simulink model "IP_Core_SS_Switch_and_PWM"  (R2018a)
settings: Solver=VariableStepAuto  StartTime=0.0  StopTime=0.05  RelTol=1e-3
values from neighbouring files (symbols this model uses):
  f_pwm_clk = 100e6    (= 100000000)    [Init_IP_Core.m]
  T_pwm_clk = 1/f_pwm_clk    (= 1e-08)    [Init_IP_Core.m]
libraries: hdlsllib x2
settings Model: Creator=BHK  LastModifiedBy=Wendel
settings OptimizationCC: BlockReduction=off  ConditionallyExecuteInputs=off  DefaultParameterBehavior=Inlined
settings DebuggingCC: AlgebraicLoopMsg=error
settings HardwareCC: ProdBitPerPointer=32  ProdBitPerSizeT=32  ProdBitPerPtrDiffT=32  ProdLargestAtomicFloat=None  ProdIntDivRoundTo=Undefined  ProdEndianess=Unspecified  ProdWordSize=32  ProdHWDeviceType=ASIC/FPGA->ASIC/FPGA  TargetBitPerPointer=64  TargetBitPerSizeT=64  TargetBitPerPtrDiffT=64  TargetLongLongMode=on  TargetIntDivRoundTo=Zero  TargetEndianess=LittleEndian  TargetWordSize=64  TargetHWDeviceType=Custom Processor->MATLAB Host Computer  ProdEqTarget=off

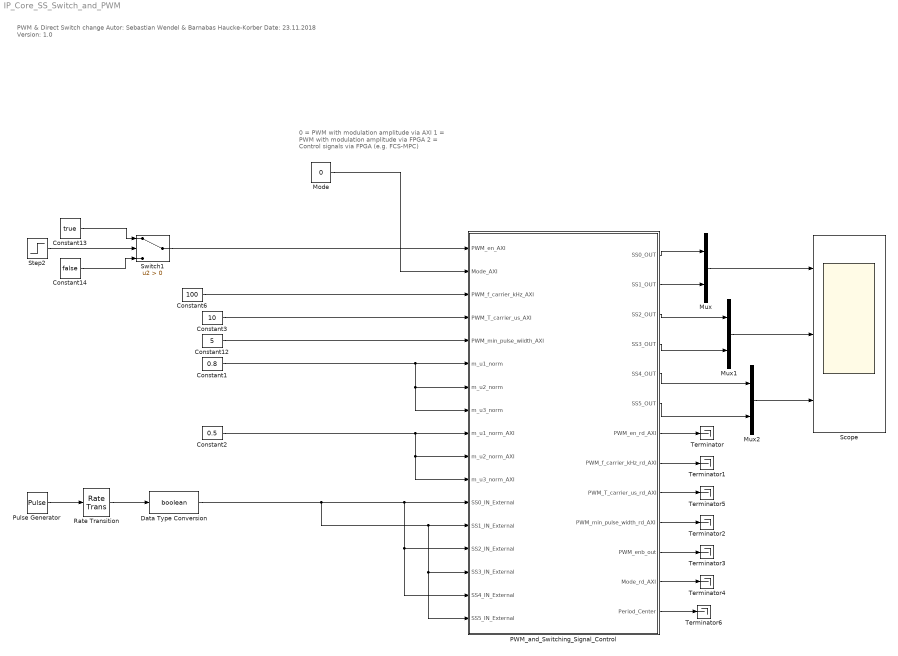
== system IP_Core_SS_Switch_and_PWM ==
  note: 0 = PWM with modulation amplitude via AXI
      | 1 = PWM with modulation amplitude via FPGA
      | 2 = Control signals via FPGA (e.g. FCS-MPC)
  note: PWM & Direct Switch change
      |
      | Autor: Sebastian Wendel & Barnabas Haucke-Korber
      | Date: 23.11.2018
      | Version: 1.0
  Constant1 : Constant  Value=0.8  OutDataTypeStr=fixdt(1,14,12)  SampleTime=T_pwm_clk
  Constant12 : Constant  Value=5  OutDataTypeStr=fixdt(0,8,0)  SampleTime=T_pwm_clk
  Constant13 : Constant  Value=true  SampleTime=T_pwm_clk
  Constant14 : Constant  Value=false  SampleTime=T_pwm_clk
  Constant2 : Constant  Value=0.5  OutDataTypeStr=fixdt(1,14,12)  SampleTime=T_pwm_clk
  Constant3 : Constant  Value=10  OutDataTypeStr=fixdt(0,8,0)  SampleTime=T_pwm_clk
  Constant6 : Constant  Value=100  OutDataTypeStr=fixdt(0,8,0)  SampleTime=T_pwm_clk
  Data Type Conversion : DataTypeConversion  OutDataTypeStr=boolean
  Mode : Constant  Value=0  OutDataTypeStr=fixdt(0,2,0)  SampleTime=T_pwm_clk
  Mux : Mux  Inputs=2
  Mux1 : Mux  Inputs=2
  Mux2 : Mux  Inputs=2
  PWM_and_Switching_Signal_Control : Subsystem  TreatAsAtomicUnit=on
  Pulse Generator : DiscretePulseGenerator  PulseType=Time based  Period=0.01  PulseWidth=5
  Rate Transition : RateTransition  OutPortSampleTime=T_pwm_clk
  Scope : Scope  NumInputPorts=3
  Step2 : Step  Time=0.002  SampleTime=T_pwm_clk
  Switch1 : Switch  Criteria=u2 > Threshold
  Terminator{,1..6} (7 alike) : Terminator
  wires:
  Step2/1 -> Switch1/2
  Constant13/1 -> Switch1/1
  Constant14/1 -> Switch1/3
  Switch1/1 -> PWM_and_Switching_Signal_Control/1(PWM_en_AXI)
  Mode/1 -> PWM_and_Switching_Signal_Control/2(Mode_AXI)
  Constant6/1 -> PWM_and_Switching_Signal_Control/3(PWM_f_carrier_kHz_AXI)
  Constant12/1 -> PWM_and_Switching_Signal_Control/5(PWM_min_pulse_wiidth_AXI)
  Constant1/1 -> PWM_and_Switching_Signal_Control/6(m_u1_norm), PWM_and_Switching_Signal_Control/8(m_u3_norm), PWM_and_Switching_Signal_Control/7(m_u2_norm)
  PWM_and_Switching_Signal_Control/7(PWM_en_rd_AXI) -> Terminator/1
  PWM_and_Switching_Signal_Control/8(PWM_f_carrier_kHz_rd_AXI) -> Terminator1/1
  PWM_and_Switching_Signal_Control/10(PWM_min_pulse_width_rd_AXI) -> Terminator2/1
  PWM_and_Switching_Signal_Control/11(PWM_enb_out) -> Terminator3/1
  PWM_and_Switching_Signal_Control/12(Mode_rd_AXI) -> Terminator4/1
  Constant2/1 -> PWM_and_Switching_Signal_Control/9(m_u1_norm_AXI), PWM_and_Switching_Signal_Control/10(m_u2_norm_AXI), PWM_and_Switching_Signal_Control/11(m_u3_norm_AXI)
  PWM_and_Switching_Signal_Control/1(SS0_OUT) -> Mux/1
  PWM_and_Switching_Signal_Control/2(SS1_OUT) -> Mux/2
  Mux/1 -> Scope/1
  PWM_and_Switching_Signal_Control/3(SS2_OUT) -> Mux1/1
  PWM_and_Switching_Signal_Control/4(SS3_OUT) -> Mux1/2
  PWM_and_Switching_Signal_Control/5(SS4_OUT) -> Mux2/1
  PWM_and_Switching_Signal_Control/6(SS5_OUT) -> Mux2/2
  Mux2/1 -> Scope/3
  Mux1/1 -> Scope/2
  Data Type Conversion/1 -> PWM_and_Switching_Signal_Control/17(SS5_IN_External), PWM_and_Switching_Signal_Control/15(SS3_IN_External), PWM_and_Switching_Signal_Control/13(SS1_IN_External), PWM_and_Switching_Signal_Control/16(SS4_IN_External), PWM_and_Switching_Signal_Control/14(SS2_IN_External), PWM_and_Switching_Signal_Control/12(SS0_IN_External)
  Constant3/1 -> PWM_and_Switching_Signal_Control/4(PWM_T_carrier_us_AXI)
  Rate Transition/1 -> Data Type Conversion/1
  Pulse Generator/1 -> Rate Transition/1
  PWM_and_Switching_Signal_Control/9(PWM_T_carrier_us_rd_AXI) -> Terminator5/1
  PWM_and_Switching_Signal_Control/13(Period_Center) -> Terminator6/1

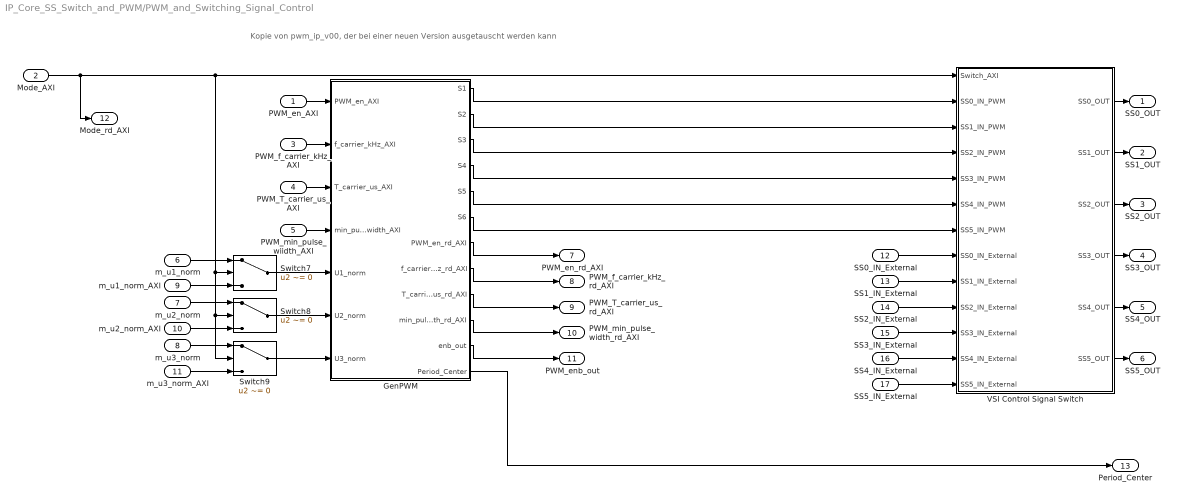
== system IP_Core_SS_Switch_and_PWM/PWM_and_Switching_Signal_Control ==
  note: Kopie von pwm_ip_v00, der bei einer neuen Version ausgetauscht werden kann
  PWM_en_AXI : Inport
  Mode_AXI : Inport  Port=2
  PWM_f_carrier_kHz_AXI : Inport  Port=3
  PWM_T_carrier_us_AXI : Inport  Port=4
  PWM_min_pulse_wiidth_AXI : Inport  Port=5
  m_u1_norm : Inport  Port=6
  m_u2_norm : Inport  Port=7
  m_u3_norm : Inport  Port=8
  m_u1_norm_AXI : Inport  Port=9
  m_u2_norm_AXI : Inport  Port=10
  m_u3_norm_AXI : Inport  Port=11
  SS0_IN_External : Inport  Port=12
  SS1_IN_External : Inport  Port=13
  SS2_IN_External : Inport  Port=14
  SS3_IN_External : Inport  Port=15
  SS4_IN_External : Inport  Port=16
  SS5_IN_External : Inport  Port=17
  GenPWM : Subsystem  TreatAsAtomicUnit=on
  Switch7 : Switch  Criteria=u2 ~= 0
  Switch8 : Switch  Criteria=u2 ~= 0
  Switch9 : Switch  Criteria=u2 ~= 0
  VSI Control Signal Switch : Subsystem
  SS0_OUT : Outport
  SS1_OUT : Outport  Port=2
  SS2_OUT : Outport  Port=3
  SS3_OUT : Outport  Port=4
  SS4_OUT : Outport  Port=5
  SS5_OUT : Outport  Port=6
  PWM_en_rd_AXI : Outport  Port=7
  PWM_f_carrier_kHz_rd_AXI : Outport  Port=8
  PWM_T_carrier_us_rd_AXI : Outport  Port=9
  PWM_min_pulse_width_rd_AXI : Outport  Port=10
  PWM_enb_out : Outport  Port=11
  Mode_rd_AXI : Outport  Port=12
  Period_Center : Outport  Port=13
  wires:
  VSI Control Signal Switch/1(SS0_OUT) -> SS0_OUT/1
  Mode_AXI/1 -> Mode_rd_AXI/1, VSI Control Signal Switch/1(Switch_AXI), Switch7/2, Switch9/2, Switch8/2
  GenPWM/4(S4) -> VSI Control Signal Switch/5(SS3_IN_PWM)
  PWM_f_carrier_kHz_AXI/1 -> GenPWM/2(f_carrier_kHz_AXI)
  GenPWM/2(S2) -> VSI Control Signal Switch/3(SS1_IN_PWM)
  SS1_IN_External/1 -> VSI Control Signal Switch/9(SS1_IN_External)
  GenPWM/3(S3) -> VSI Control Signal Switch/4(SS2_IN_PWM)
  GenPWM/5(S5) -> VSI Control Signal Switch/6(SS4_IN_PWM)
  GenPWM/6(S6) -> VSI Control Signal Switch/7(SS5_IN_PWM)
  VSI Control Signal Switch/6(SS5_OUT) -> SS5_OUT/1
  GenPWM/1(S1) -> VSI Control Signal Switch/2(SS0_IN_PWM)
  GenPWM/11(enb_out) -> PWM_enb_out/1
  VSI Control Signal Switch/3(SS2_OUT) -> SS2_OUT/1
  SS3_IN_External/1 -> VSI Control Signal Switch/11(SS3_IN_External)
  SS0_IN_External/1 -> VSI Control Signal Switch/8(SS0_IN_External)
  VSI Control Signal Switch/2(SS1_OUT) -> SS1_OUT/1
  SS4_IN_External/1 -> VSI Control Signal Switch/12(SS4_IN_External)
  PWM_en_AXI/1 -> GenPWM/1(PWM_en_AXI)
  SS5_IN_External/1 -> VSI Control Signal Switch/13(SS5_IN_External)
  VSI Control Signal Switch/5(SS4_OUT) -> SS4_OUT/1
  PWM_min_pulse_wiidth_AXI/1 -> GenPWM/4(min_pulse_width_AXI)
  SS2_IN_External/1 -> VSI Control Signal Switch/10(SS2_IN_External)
  VSI Control Signal Switch/4(SS3_OUT) -> SS3_OUT/1
  Switch9/1 -> GenPWM/7(U3_norm)
  m_u1_norm_AXI/1 -> Switch7/3
  m_u1_norm/1 -> Switch7/1
  m_u2_norm/1 -> Switch8/1
  m_u2_norm_AXI/1 -> Switch8/3
  m_u3_norm/1 -> Switch9/1
  m_u3_norm_AXI/1 -> Switch9/3
  GenPWM/7(PWM_en_rd_AXI) -> PWM_en_rd_AXI/1
  GenPWM/8(f_carrier_kHz_rd_AXI) -> PWM_f_carrier_kHz_rd_AXI/1
  GenPWM/10(min_pulse_width_rd_AXI) -> PWM_min_pulse_width_rd_AXI/1
  GenPWM/9(T_carrier_us_rd_AXI) -> PWM_T_carrier_us_rd_AXI/1
  Switch8/1 -> GenPWM/6(U2_norm)
  Switch7/1 -> GenPWM/5(U1_norm)
  PWM_T_carrier_us_AXI/1 -> GenPWM/3(T_carrier_us_AXI)
  GenPWM/12(Period_Center) -> Period_Center/1

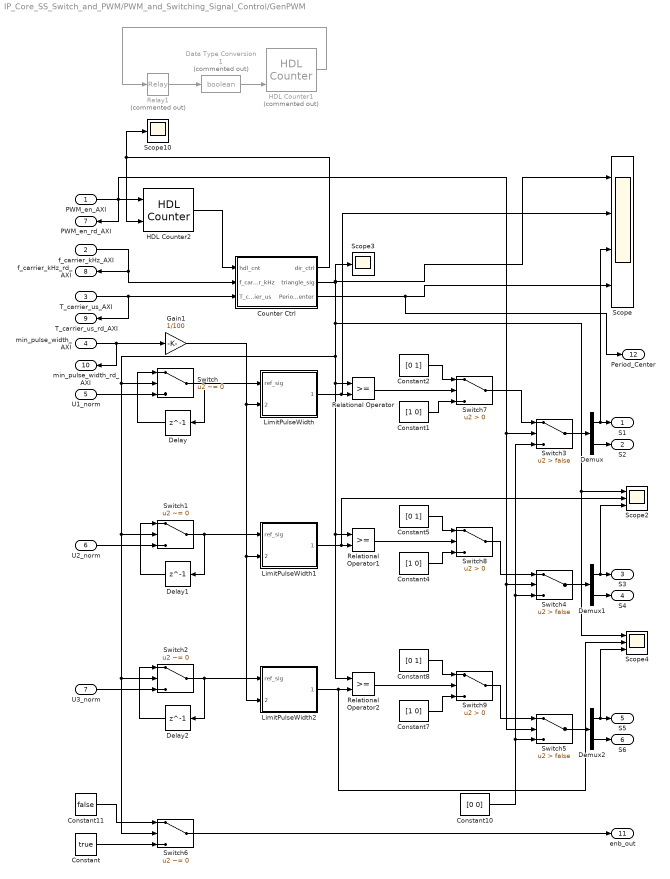
== system IP_Core_SS_Switch_and_PWM/PWM_and_Switching_Signal_Control/GenPWM ==
  PWM_en_AXI : Inport
  f_carrier_kHz_AXI : Inport  Port=2
  T_carrier_us_AXI : Inport  Port=3
  min_pulse_width_AXI : Inport  Port=4
  U1_norm : Inport  Port=5
  U2_norm : Inport  Port=6
  U3_norm : Inport  Port=7
  Constant : Constant  Value=true  SampleTime=T_pwm_clk
  Constant1 : Constant  Value=[1 0]  OutDataTypeStr=fixdt(0,1,0)  SampleTime=T_pwm_clk
  Constant10 : Constant  Value=[0 0]  OutDataTypeStr=fixdt(0,1,0)  SampleTime=T_pwm_clk
  Constant11 : Constant  Value=false  SampleTime=T_pwm_clk
  Constant2 : Constant  Value=[0 1]  OutDataTypeStr=fixdt(0,1,0)  SampleTime=T_pwm_clk
  Constant4 : Constant  Value=[1 0]  OutDataTypeStr=fixdt(0,1,0)  SampleTime=T_pwm_clk
  Constant5 : Constant  Value=[0 1]  OutDataTypeStr=fixdt(0,1,0)  SampleTime=T_pwm_clk
  Constant7 : Constant  Value=[1 0]  OutDataTypeStr=fixdt(0,1,0)  SampleTime=T_pwm_clk
  Constant8 : Constant  Value=[0 1]  OutDataTypeStr=fixdt(0,1,0)  SampleTime=T_pwm_clk
  Counter Ctrl : Subsystem
  Data Type Conversion1 : DataTypeConversion  Commented=on  OutDataTypeStr=boolean
  Delay : Delay  DelayLength=1
  Delay1 : Delay  DelayLength=1
  Delay2 : Delay  DelayLength=1
  Demux : Demux  Outputs=2
  Demux1 : Demux  Outputs=2
  Demux2 : Demux  Outputs=2
  Gain1 : Gain  Gain=1/100  OutDataTypeStr=fixdt(1,18,10)
  HDL Counter1 : hdlsllib/Sources/HDL Counter  Commented=on  CountType=Free running  CountInit=0  CountStep=1  CountMax=100  CountFromType=Initial value  CountFrom=0  CountResetPort=on  CountLoadPort=off  CountEnbPort=on  CountDirPort=on  CountDataType=Signed  CountWordLen=8  CountFracLen=0  CountSampTime=Ts
      settings: SourceProductBaseCode=HD
  HDL Counter2 : hdlsllib/Sources/HDL Counter  CountType=Free running  CountInit=0  CountStep=1  CountMax=100  CountFromType=Initial value  CountFrom=0  CountResetPort=off  CountLoadPort=off  CountEnbPort=on  CountDirPort=on  CountDataType=Unsigned  CountWordLen=20  CountFracLen=0  CountSampTime=1
      settings: SourceProductBaseCode=HD
  LimitPulseWidth : Subsystem
  LimitPulseWidth1 : Subsystem
  LimitPulseWidth2 : Subsystem
  Relational Operator : RelationalOperator  OutDataTypeStr=boolean  RndMeth=Nearest
  Relational Operator1 : RelationalOperator  OutDataTypeStr=boolean  RndMeth=Nearest
  Relational Operator2 : RelationalOperator  OutDataTypeStr=boolean  RndMeth=Nearest
  Relay1 : Relay  Commented=on  OnSwitchValue=100  OffSwitchValue=0  OnOutputValue=0  OffOutputValue=1
  Scope : Scope  NumInputPorts=4
  Scope10 : Scope
  Scope2 : Scope  NumInputPorts=3
  Scope3 : Scope
  Scope4 : Scope  NumInputPorts=3
  Switch{,1..2,6} (4 alike) : Switch  Criteria=u2 ~= 0
  Switch3 : Switch  Criteria=u2 > Threshold  Threshold=false
  Switch4 : Switch  Criteria=u2 > Threshold  Threshold=false
  Switch5 : Switch  Criteria=u2 > Threshold  Threshold=false
  Switch7 : Switch  Criteria=u2 > Threshold
  Switch8 : Switch  Criteria=u2 > Threshold
  Switch9 : Switch  Criteria=u2 > Threshold
  S1 : Outport
  S2 : Outport  Port=2
  S3 : Outport  Port=3
  S4 : Outport  Port=4
  S5 : Outport  Port=5
  S6 : Outport  Port=6
  PWM_en_rd_AXI : Outport  Port=7
  f_carrier_kHz_rd_AXI : Outport  Port=8
  T_carrier_us_rd_AXI : Outport  Port=9
  min_pulse_width_rd_AXI : Outport  Port=10
  enb_out : Outport  Port=11
  Period_Center : Outport  Port=12
  wires:
  Constant7/1 -> Switch9/3
  Demux2/2 -> S6/1
  Constant8/1 -> Switch9/1
  Relational Operator2/1 -> Switch9/2
  Switch9/1 -> Switch5/1
  Demux/2 -> S2/1
  Relational Operator/1 -> Switch7/2
  Demux1/2 -> S4/1
  Constant5/1 -> Switch8/1
  Relational Operator1/1 -> Switch8/2
  Constant4/1 -> Switch8/3
  Constant1/1 -> Switch7/3
  Constant2/1 -> Switch7/1
  LimitPulseWidth/1(ref_sig_limit) -> Scope/2, Relational Operator/2
  LimitPulseWidth1/1(ref_sig_limit) -> Scope2/2, Relational Operator1/2
  LimitPulseWidth2/1(ref_sig_limit) -> Scope4/2, Relational Operator2/2
  Counter Ctrl/2(triangle_sig) -> Relational Operator2/1, Relational Operator1/1, Relational Operator/1, Switch6/2, Switch2/2, Switch1/2, Switch/2, Scope4/1, Scope2/1, Scope3/1, Scope/1
  PWM_en_AXI/1 -> Switch3/2, Switch5/2, Switch4/2, PWM_en_rd_AXI/1, HDL Counter2/1
  Delay/1 -> Switch/1
  Delay1/1 -> Switch1/1
  Delay2/1 -> Switch2/1
  Switch5/1 -> Demux2/1
  Switch8/1 -> Switch4/1
  Switch4/1 -> Demux1/1
  Switch3/1 -> Demux/1
  Constant10/1 -> Switch5/3, Switch4/3, Switch3/3
  U1_norm/1 -> Switch/3
  U3_norm/1 -> Switch2/3
  U2_norm/1 -> Switch1/3
  Counter Ctrl/1(dir_ctrl) -> HDL Counter2/2, Scope10/1
  HDL Counter2/1 -> Counter Ctrl/1(hdl_cnt)
  f_carrier_kHz_AXI/1 -> f_carrier_kHz_rd_AXI/1, Counter Ctrl/2(f_carrier_kHz)
  Relay1/1 -> Data Type Conversion1/1
  Data Type Conversion1/1 -> HDL Counter1/3
  HDL Counter1/1 -> Relay1/1
  Switch/1 -> LimitPulseWidth/1(ref_sig), Delay/1
  Switch1/1 -> LimitPulseWidth1/1(ref_sig), Delay1/1
  Switch2/1 -> LimitPulseWidth2/1(ref_sig), Delay2/1
  min_pulse_width_AXI/1 -> Gain1/1, min_pulse_width_rd_AXI/1
  Demux/1 -> Scope/3, S1/1
  Switch6/1 -> enb_out/1
  Constant11/1 -> Switch6/1
  Constant/1 -> Switch6/3
  Demux1/1 -> Scope2/3, S3/1
  Demux2/1 -> Scope4/3, S5/1
  T_carrier_us_AXI/1 -> T_carrier_us_rd_AXI/1, Counter Ctrl/3(T_carrier_us)
  Switch7/1 -> Switch3/1
  Gain1/1 -> LimitPulseWidth/2(min_pulse_width), LimitPulseWidth2/2(min_pulse_width), LimitPulseWidth1/2(min_pulse_width)
  Counter Ctrl/3(Period_Center) -> Period_Center/1, Scope/4

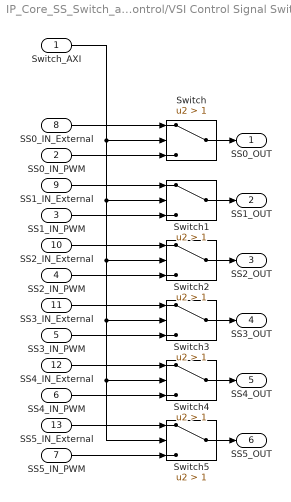
== system IP_Core_SS_Switch_and_PWM/PWM_and_Switching_Signal_Control/VSI Control Signal Switch ==
  Switch_AXI : Inport
  SS0_IN_PWM : Inport  Port=2
  SS1_IN_PWM : Inport  Port=3
  SS2_IN_PWM : Inport  Port=4
  SS3_IN_PWM : Inport  Port=5
  SS4_IN_PWM : Inport  Port=6
  SS5_IN_PWM : Inport  Port=7
  SS0_IN_External : Inport  Port=8
  SS1_IN_External : Inport  Port=9
  SS2_IN_External : Inport  Port=10
  SS3_IN_External : Inport  Port=11
  SS4_IN_External : Inport  Port=12
  SS5_IN_External : Inport  Port=13
  Switch{,1..5} (6 alike) : Switch  Criteria=u2 > Threshold  Threshold=1
  SS0_OUT : Outport
  SS1_OUT : Outport  Port=2
  SS2_OUT : Outport  Port=3
  SS3_OUT : Outport  Port=4
  SS4_OUT : Outport  Port=5
  SS5_OUT : Outport  Port=6
  wires:
  Switch_AXI/1 -> Switch4/2, Switch5/2, Switch3/2, Switch2/2, Switch1/2, Switch/2
  Switch5/1 -> SS5_OUT/1
  Switch/1 -> SS0_OUT/1
  Switch3/1 -> SS3_OUT/1
  Switch2/1 -> SS2_OUT/1
  Switch1/1 -> SS1_OUT/1
  Switch4/1 -> SS4_OUT/1
  SS0_IN_PWM/1 -> Switch/3
  SS0_IN_External/1 -> Switch/1
  SS1_IN_External/1 -> Switch1/1
  SS1_IN_PWM/1 -> Switch1/3
  SS2_IN_External/1 -> Switch2/1
  SS2_IN_PWM/1 -> Switch2/3
  SS3_IN_External/1 -> Switch3/1
  SS3_IN_PWM/1 -> Switch3/3
  SS4_IN_External/1 -> Switch4/1
  SS4_IN_PWM/1 -> Switch4/3
  SS5_IN_External/1 -> Switch5/1
  SS5_IN_PWM/1 -> Switch5/3

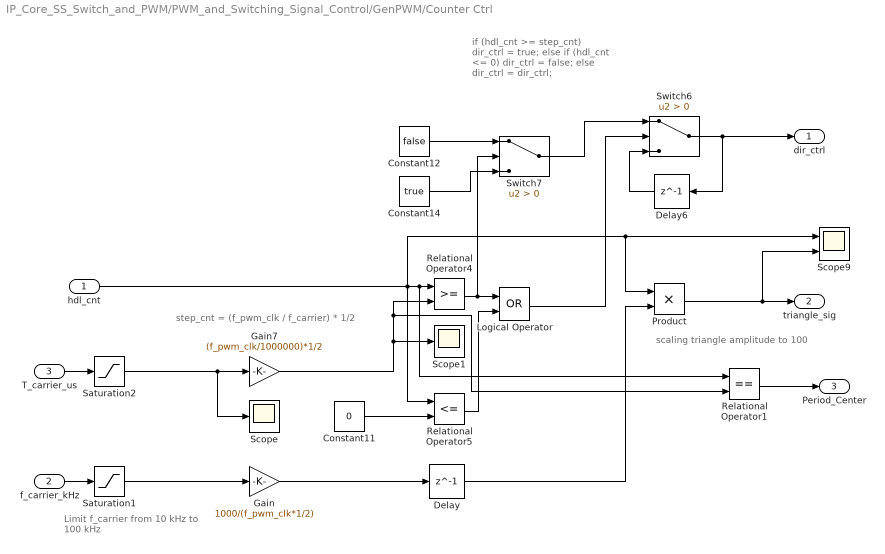
== system IP_Core_SS_Switch_and_PWM/PWM_and_Switching_Signal_Control/GenPWM/Counter Ctrl ==
  note: if (hdl_cnt >= step_cnt)
      | 	dir_ctrl = true;
      | else if (hdl_cnt <= 0)
      | 	dir_ctrl = false;
      | else
      | 	dir_ctrl = dir_ctrl;
  note: step_cnt = (f_pwm_clk / f_carrier) * 1/2
  note: scaling triangle amplitude to 100
  note: Limit f_carrier from
      | 10 kHz to 100 kHz
  hdl_cnt : Inport
  f_carrier_kHz : Inport  Port=2
  T_carrier_us : Inport  Port=3
  Constant11 : Constant  Value=0  OutDataTypeStr=fixdt(0,20,0)  SampleTime=T_pwm_clk
  Constant12 : Constant  Value=false  SampleTime=T_pwm_clk
  Constant14 : Constant  Value=true  SampleTime=T_pwm_clk
  Delay : Delay  DelayLength=1
  Delay6 : Delay  DelayLength=1
  Gain : Gain  Gain=1000/(f_pwm_clk*1/2)  OutDataTypeStr=fixdt(0,18,19)
  Gain7 : Gain  Gain=(f_pwm_clk/1000000)*1/2  OutDataTypeStr=fixdt(0,20,0)
  Logical Operator : Logic  Operator=OR  AllPortsSameDT=off  OutDataTypeStr=boolean
  Product : Product  OutDataTypeStr=fixdt(0,18,10)
  Relational Operator1 : RelationalOperator  Operator===  OutDataTypeStr=boolean  RndMeth=Nearest
  Relational Operator4 : RelationalOperator  OutDataTypeStr=boolean  RndMeth=Nearest
  Relational Operator5 : RelationalOperator  Operator=<=  OutDataTypeStr=boolean  RndMeth=Nearest
  Saturation1 : Saturate  UpperLimit=100  LowerLimit=10
  Saturation2 : Saturate  UpperLimit=100  LowerLimit=10
  Scope : Scope
  Scope1 : Scope
  Scope9 : Scope  NumInputPorts=2
  Switch6 : Switch  Criteria=u2 > Threshold
  Switch7 : Switch  Criteria=u2 > Threshold
  dir_ctrl : Outport
  triangle_sig : Outport  Port=2
  Period_Center : Outport  Port=3
  wires:
  hdl_cnt/1 -> Product/1, Scope9/1, Relational Operator1/1, Relational Operator4/1, Relational Operator5/1
  Switch6/1 -> Delay6/1, dir_ctrl/1
  Relational Operator4/1 -> Switch7/2, Logical Operator/1
  Relational Operator5/1 -> Logical Operator/2
  Constant11/1 -> Relational Operator5/2
  Logical Operator/1 -> Switch6/2
  Switch7/1 -> Switch6/1
  Constant12/1 -> Switch7/1
  Constant14/1 -> Switch7/3
  Delay6/1 -> Switch6/3
  f_carrier_kHz/1 -> Saturation1/1
  Saturation2/1 -> Scope/1, Gain7/1
  T_carrier_us/1 -> Saturation2/1
  Gain7/1 -> Scope1/1, Relational Operator1/2, Relational Operator4/2
  Saturation1/1 -> Gain/1
  Product/1 -> triangle_sig/1, Scope9/2
  Gain/1 -> Delay/1
  Delay/1 -> Product/2
  Relational Operator1/1 -> Period_Center/1

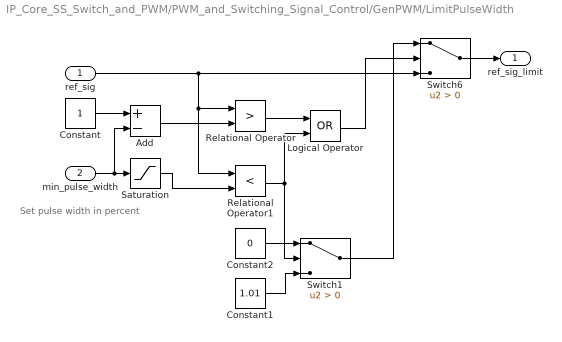
== system IP_Core_SS_Switch_and_PWM/PWM_and_Switching_Signal_Control/GenPWM/LimitPulseWidth ==
  note: Set pulse width in percent
  ref_sig : Inport
  min_pulse_width : Inport  Port=2
  Add : Sum  Inputs=+-  OutDataTypeStr=fixdt(0,18,10)
  Constant : Constant  OutDataTypeStr=fixdt(1,18,10)  SampleTime=T_pwm_clk
  Constant1 : Constant  Value=1.01  OutDataTypeStr=fixdt(0,18,10)  SampleTime=T_pwm_clk
  Constant2 : Constant  Value=0  OutDataTypeStr=fixdt(0,18,10)  SampleTime=T_pwm_clk
  Logical Operator : Logic  Operator=OR  AllPortsSameDT=off  OutDataTypeStr=boolean
  Relational Operator : RelationalOperator  Operator=>  OutDataTypeStr=boolean  RndMeth=Nearest
  Relational Operator1 : RelationalOperator  Operator=<  OutDataTypeStr=boolean  RndMeth=Nearest
  Saturation : Saturate  UpperLimit=1  LowerLimit=0  OutDataTypeStr=fixdt(0,18,10)
  Switch1 : Switch  Criteria=u2 > Threshold
  Switch6 : Switch  Criteria=u2 > Threshold
  ref_sig_limit : Outport
  wires:
  Constant/1 -> Add/1
  min_pulse_width/1 -> Add/2, Saturation/1
  Add/1 -> Relational Operator/2
  ref_sig/1 -> Switch6/3, Relational Operator/1, Relational Operator1/1
  Relational Operator/1 -> Logical Operator/1
  Relational Operator1/1 -> Logical Operator/2, Switch1/2
  Logical Operator/1 -> Switch6/2
  Constant1/1 -> Switch1/3
  Switch1/1 -> Switch6/1
  Constant2/1 -> Switch1/1
  Switch6/1 -> ref_sig_limit/1
  Saturation/1 -> Relational Operator1/2

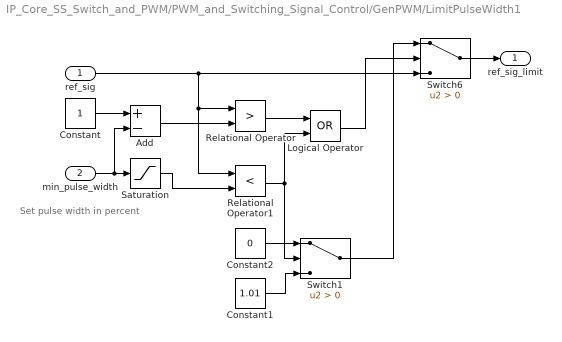
== system IP_Core_SS_Switch_and_PWM/PWM_and_Switching_Signal_Control/GenPWM/LimitPulseWidth1 ==
  note: Set pulse width in percent
  ref_sig : Inport
  min_pulse_width : Inport  Port=2
  Add : Sum  Inputs=+-  OutDataTypeStr=fixdt(0,18,10)
  Constant : Constant  OutDataTypeStr=fixdt(1,18,10)  SampleTime=T_pwm_clk
  Constant1 : Constant  Value=1.01  OutDataTypeStr=fixdt(0,18,10)  SampleTime=T_pwm_clk
  Constant2 : Constant  Value=0  OutDataTypeStr=fixdt(0,18,10)  SampleTime=T_pwm_clk
  Logical Operator : Logic  Operator=OR  AllPortsSameDT=off  OutDataTypeStr=boolean
  Relational Operator : RelationalOperator  Operator=>  OutDataTypeStr=boolean  RndMeth=Nearest
  Relational Operator1 : RelationalOperator  Operator=<  OutDataTypeStr=boolean  RndMeth=Nearest
  Saturation : Saturate  UpperLimit=1  LowerLimit=0  OutDataTypeStr=fixdt(0,18,10)
  Switch1 : Switch  Criteria=u2 > Threshold
  Switch6 : Switch  Criteria=u2 > Threshold
  ref_sig_limit : Outport
  wires:
  Constant/1 -> Add/1
  min_pulse_width/1 -> Add/2, Saturation/1
  Add/1 -> Relational Operator/2
  ref_sig/1 -> Switch6/3, Relational Operator/1, Relational Operator1/1
  Relational Operator/1 -> Logical Operator/1
  Relational Operator1/1 -> Logical Operator/2, Switch1/2
  Logical Operator/1 -> Switch6/2
  Constant1/1 -> Switch1/3
  Switch1/1 -> Switch6/1
  Constant2/1 -> Switch1/1
  Switch6/1 -> ref_sig_limit/1
  Saturation/1 -> Relational Operator1/2

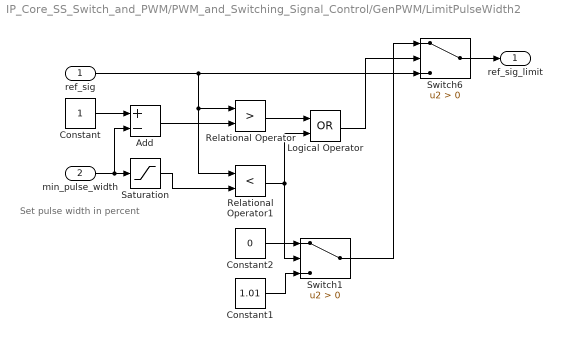
== system IP_Core_SS_Switch_and_PWM/PWM_and_Switching_Signal_Control/GenPWM/LimitPulseWidth2 ==
  note: Set pulse width in percent
  ref_sig : Inport
  min_pulse_width : Inport  Port=2
  Add : Sum  Inputs=+-  OutDataTypeStr=fixdt(0,18,10)
  Constant : Constant  OutDataTypeStr=fixdt(1,18,10)  SampleTime=T_pwm_clk
  Constant1 : Constant  Value=1.01  OutDataTypeStr=fixdt(0,18,10)  SampleTime=T_pwm_clk
  Constant2 : Constant  Value=0  OutDataTypeStr=fixdt(0,18,10)  SampleTime=T_pwm_clk
  Logical Operator : Logic  Operator=OR  AllPortsSameDT=off  OutDataTypeStr=boolean
  Relational Operator : RelationalOperator  Operator=>  OutDataTypeStr=boolean  RndMeth=Nearest
  Relational Operator1 : RelationalOperator  Operator=<  OutDataTypeStr=boolean  RndMeth=Nearest
  Saturation : Saturate  UpperLimit=1  LowerLimit=0  OutDataTypeStr=fixdt(0,18,10)
  Switch1 : Switch  Criteria=u2 > Threshold
  Switch6 : Switch  Criteria=u2 > Threshold
  ref_sig_limit : Outport
  wires:
  Constant/1 -> Add/1
  min_pulse_width/1 -> Add/2, Saturation/1
  Add/1 -> Relational Operator/2
  ref_sig/1 -> Switch6/3, Relational Operator/1, Relational Operator1/1
  Relational Operator/1 -> Logical Operator/1
  Relational Operator1/1 -> Logical Operator/2, Switch1/2
  Logical Operator/1 -> Switch6/2
  Constant1/1 -> Switch1/3
  Switch1/1 -> Switch6/1
  Constant2/1 -> Switch1/1
  Switch6/1 -> ref_sig_limit/1
  Saturation/1 -> Relational Operator1/2
